simulink model "Orbit_Propagator_Model"  (R2024a)
settings: Solver=VariableStepAuto  StartTime=0.0  StopTime=10.0  RelTol=1e-3
undefined symbols (not defined in the file or in its folder): IAU
libraries: aerolibtransform2 x1
settings Model: Creator=hendr  LastModifiedBy=hendr

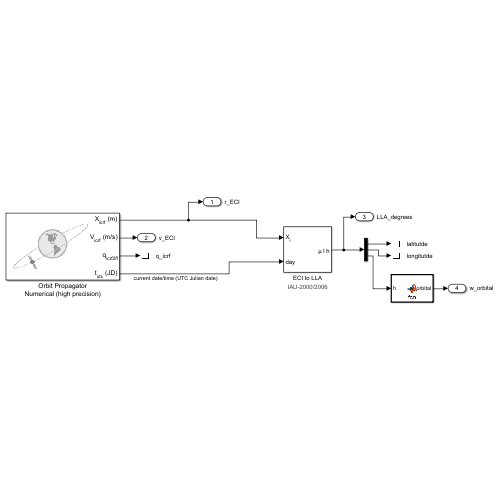
[thumbnail: Simulink's stored preview of the top-level diagram]
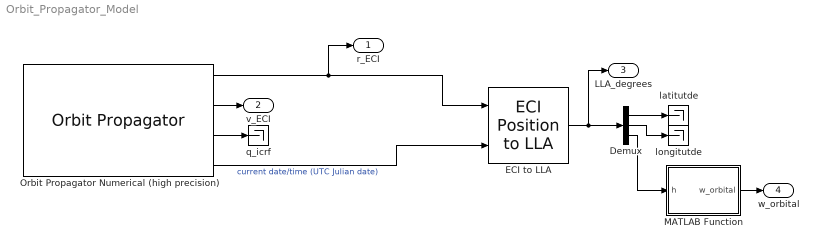
== system Orbit_Propagator_Model ==
  Demux : Demux  Outputs=3
  ECI to LLA : aerolibtransform2/ECI Position to LLA  red=IAU-2000/2006  year=2013  month=January  day=1  hour=0  min=0  sec=0  deltaT=Day  errorflag=Error  extraparamflag=off  eunits=Metric (MKS)  earthmodel=WGS84  flat=1/298.257223563  eqradius=6378137
      settings: AttributesFormatString=%<red>
  MATLAB Function : MATLAB Function  TreatAsAtomicUnit=on
  Orbit Propagator Numerical (high precision) : OrbitPropagator  propagator=Numerical (high precision)  semiMajorAxis=orbit.a  eccentricity=orbit.e  inclination=orbit.i  raan=orbit.Omega  argPeriapsis=orbit.omega  trueAnomaly=orbit.M0  inertialPosition=[3649700.0 3308200.0 -4676600.0]  inertialVelocity=[-2750.8 6666.4 2573.4]  fixedPosition=[-4142689.0 -2676864.7 -4669861.6]  fixedVelocity=[1452.7 -6720.7 2568.1]  customR=3396200  customMu=4.305e13  customJ2=1.0826269e-03  customOmega=4.06125949e-3  outputTransform=on
  latitutde : Terminator
  longitutde : Terminator
  q_icrf : Terminator
  r_ECI : Outport
  v_ECI : Outport  Port=2
  LLA_degrees : Outport  Port=3
  w_orbital : Outport  Port=4
  wires:
  Orbit Propagator Numerical (high precision)/3 -> q_icrf/1
  Orbit Propagator Numerical (high precision)/4 -> ECI to LLA/2  "current date/time (UTC Julian date)"
  Orbit Propagator Numerical (high precision)/1 -> ECI to LLA/1, r_ECI/1
  Orbit Propagator Numerical (high precision)/2 -> v_ECI/1
  ECI to LLA/1 -> Demux/1, LLA_degrees/1
  MATLAB Function/1(w_orbital) -> w_orbital/1
  Demux/2 -> longitutde/1
  Demux/3 -> MATLAB Function/1(h)
  Demux/1 -> latitutde/1

== matlab function Orbit_Propagator_Model/MATLAB Function ==
  data: h input; w_orbital output
function w_orbital = fcn(h)


mu = 398600.4418e9; % m^3/s^2
Re = 6378000; % m
w_orbital = sqrt(mu/(Re+h)^3); % rad/s

end
